simulink model "p_controller"  (R2022a)
settings: Solver=VariableStepAuto  StartTime=0.0  StopTime=10.0  RelTol=1e-3
settings Model: Creator=Laptop-Academy.com  LastModifiedBy=Laptop-Academy.com

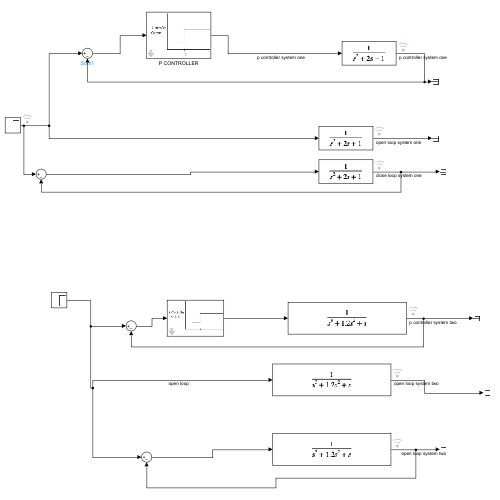
[thumbnail: Simulink's stored preview of the top-level diagram]
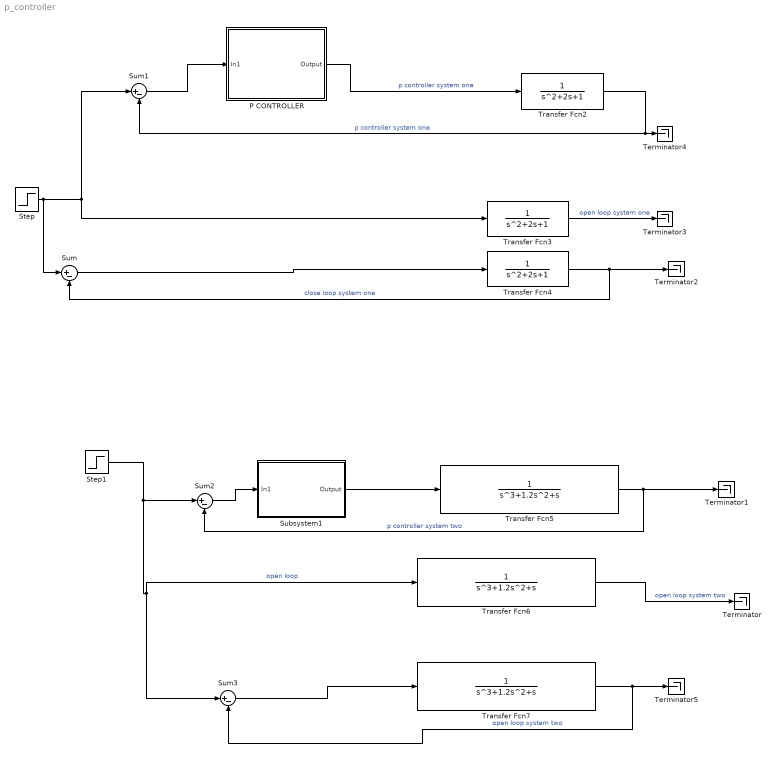
== system p_controller ==
  P CONTROLLER : Subsystem  mask{p=0}
      mask prompts: p "p gain (p)"
      mask Display: image("F:\os_academy_labs\pid_controller\media\p_controller.jpg");
  Step : Step  SampleTime=0
  Step1 : Step  SampleTime=0
  Subsystem1 : Subsystem  mask{p=0}
      mask prompts: p "propotional gain (p)"
      mask Display: image("F:\os_academy_labs\pid_controller\media\p_controller.jpg");
  Sum{,1..3} (4 alike) : Sum  Inputs=|+-
  Terminator{,1..5} (6 alike) : Terminator
  Transfer Fcn2 : TransferFcn
  Transfer Fcn3 : TransferFcn
  Transfer Fcn4 : TransferFcn
  Transfer Fcn5 : TransferFcn  Denominator=[1 1.2 1 0]
  Transfer Fcn6 : TransferFcn  Denominator=[1 1.2 1 0]
  Transfer Fcn7 : TransferFcn  Denominator=[1 1.2 1 0]
  wires:
  Transfer Fcn4/1 -> Terminator2/1, Sum/2  "close loop system one"
  Transfer Fcn2/1 -> Sum1/2, Terminator4/1  "p controller system one"
  Transfer Fcn3/1 -> Terminator3/1  "open loop system one"
  Transfer Fcn6/1 -> Terminator/1  "open loop system two"
  Subsystem1/1(Output) -> Transfer Fcn5/1
  Step1/1 -> Sum2/1, Sum3/1, Transfer Fcn6/1  "open loop"
  Transfer Fcn5/1 -> Sum2/2, Terminator1/1  "p controller system two"
  Transfer Fcn7/1 -> Sum3/2, Terminator5/1  "open loop system two"
  Sum3/1 -> Transfer Fcn7/1
  P CONTROLLER/1(Output) -> Transfer Fcn2/1  "p controller system one"
  Sum/1 -> Transfer Fcn4/1
  Step/1 -> Sum1/1, Transfer Fcn3/1, Sum/1
  Sum1/1 -> P CONTROLLER/1(In1)
  Sum2/1 -> Subsystem1/1(In1)

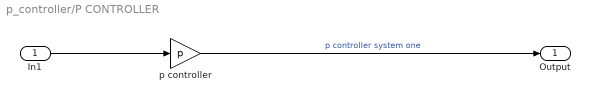
== system p_controller/P CONTROLLER ==
  In1 : Inport
  p controller : Gain  Gain=p
  Output : Outport
  wires:
  p controller/1 -> Output/1  "p controller system one"
  In1/1 -> p controller/1

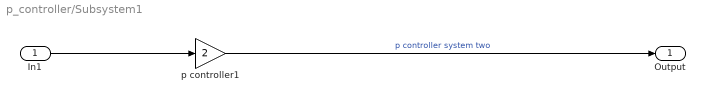
== system p_controller/Subsystem1 ==
  In1 : Inport
  p controller1 : Gain  Gain=2
  Output : Outport
  wires:
  p controller1/1 -> Output/1  "p controller system two"
  In1/1 -> p controller1/1
